simulink model "lab3_1"  (R2021a)
settings: Solver=VariableStepAuto  StartTime=0.0  StopTime=30.0  RelTol=1e-10  AbsTol=1e-10
values from neighbouring files (symbols this model uses):
  dbar = g*sin(theta)    [lab3.m]
  vdes = 14    [lab3.m]
libraries: cstblocks x2
settings Model: Creator=markalex  LastModifiedBy=markalex

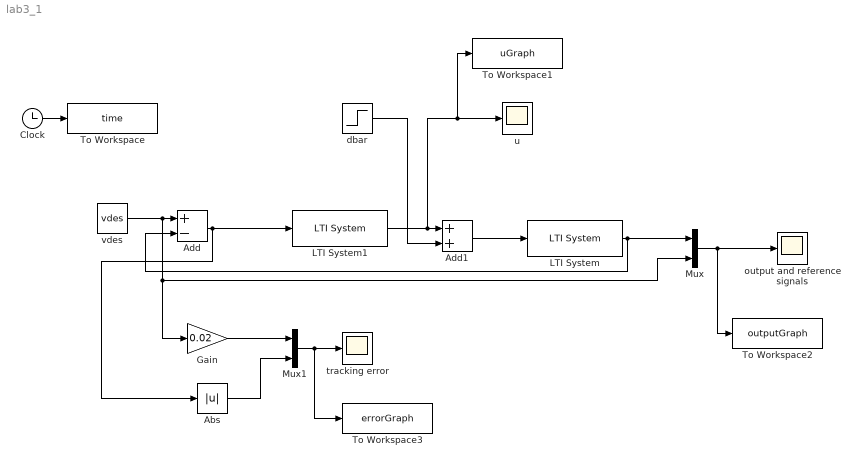
== system lab3_1 ==
  Abs : Abs
  Add : Sum  Inputs=+-
  Add1 : Sum
  Clock : Clock
  Gain : Gain  Gain=0.02
  LTI System : cstblocks/LTI System  sys=G  IC=[]
  LTI System1 : cstblocks/LTI System  sys=C  IC=[]
  Mux : Mux  Inputs=2
  Mux1 : Mux  Inputs=2
  To Workspace : ToWorkspace  VariableName=time  SampleTime=1e-3
  To Workspace1 : ToWorkspace  VariableName=uGraph  SampleTime=1e-3
  To Workspace2 : ToWorkspace  VariableName=outputGraph  SampleTime=1e-3
  To Workspace3 : ToWorkspace  VariableName=errorGraph  SampleTime=1e-3
  dbar : Step  Time=15  After=dbar  SampleTime=0
  output and reference signals : Scope
  tracking error : Scope
  u : Scope
  vdes : Constant  Value=vdes
  wires:
  vdes/1 -> Gain/1, Mux/2, Add/1
  Add/1 -> Abs/1, LTI System1/1
  LTI System1/1 -> To Workspace1/1, u/1, Add1/1
  Add1/1 -> LTI System/1
  LTI System/1 -> Add/2, Mux/1
  Mux/1 -> To Workspace2/1, output and reference signals/1
  Gain/1 -> Mux1/1
  Mux1/1 -> tracking error/1, To Workspace3/1
  Abs/1 -> Mux1/2
  dbar/1 -> Add1/2
  Clock/1 -> To Workspace/1
